simulink model "zoh"  (R2015b)
settings: Solver=VariableStepAuto  StartTime=0.0  StopTime=30.0  RelTol=1e-3
settings Model: Creator=ovi  LastModifiedBy=ovi

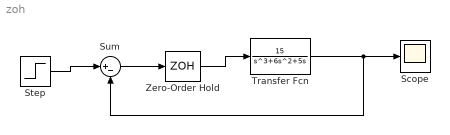
== system zoh ==
  Scope : Scope
  Step : Step  SampleTime=0
  Sum : Sum  Inputs=|+-
  Transfer Fcn : TransferFcn  Numerator=[15]  Denominator=[1 6 5 0]
  Zero-Order Hold : ZeroOrderHold  SampleTime=0.01
  wires:
  Step/1 -> Sum/1
  Sum/1 -> Zero-Order Hold/1
  Zero-Order Hold/1 -> Transfer Fcn/1
  Transfer Fcn/1 -> Sum/2, Scope/1
